simulink model "carsim_experiment_commai"  (R2017a)
settings: Solver=ode45  StartTime=0  StopTime=200  FixedStep=0.002  RelTol=1e-3  AbsTol=1e-6
PreLoadFcn:
  | addpath C:\MKZ
  | bus_definitions
libraries: Solver_SF x1
settings Model: ExtModeTrigMode=oneshot  ExtModeArmWhenConnect=off  Creator=ywata  LastModifiedBy=User
settings DataIOCC: SaveFormat=Array  SignalLoggingName=sigsOut
settings OptimizationCC: BlockReduction=off  BooleanDataType=off  LifeSpan=inf
settings DebuggingCC: SaveWithParameterizedLinksMsg=none  UnderspecifiedInitializationDetection=Classic  MergeDetectMultiDrivingBlocksExec=none  SignalResolutionControl=TryResolveAllWithWarning  MultiTaskDSMMsg=warning  MultiTaskCondExecSysMsg=none  FcnCallInpInsideContextMsg=warning  StateNameClashWarn=warning  SFUnexpectedBacktrackingDiag=warning  SFNoUnconditionalDefaultTransitionDiag=warning  SFExecutionAtInitializationDiag=none
settings HardwareCC: ProdBitPerPointer=32  ProdBitPerSizeT=32  ProdBitPerPtrDiffT=32  ProdLargestAtomicFloat=None  ProdIntDivRoundTo=Undefined  ProdEndianess=Unspecified  ProdWordSize=32  ProdHWDeviceType=32-bit Generic  TargetBitPerPointer=64  TargetBitPerSizeT=64  TargetBitPerPtrDiffT=64  TargetLongLongMode=on  TargetIntDivRoundTo=Zero  TargetEndianess=LittleEndian  TargetWordSize=64  TargetHWDeviceType=MATLAB Host  ProdEqTarget=off
settings ModelReferenceCC: UpdateModelReferenceTargets=Force  ModelReferenceNumInstancesAllowed=Single  PropagateSignalLabelsOutOfModel=off
settings ModelReferenceCC: ModelDependencies=|
  | lk_pcis_controller.m
  | road.m
settings RTWCC: TemplateMakefile=grt_vc.tmf
settings GRTTargetCC: TargetFcnLib=ansi_tfl_tmw.mat  TargetLangStandard=C89/C90 (ANSI)  GeneratePreprocessorConditionals=Disable all  CombineOutputUpdateFcns=off  GRTInterface=on
settings ConfigComp: CovMetricSettings=dw  CovHtmlReporting=on  CovSaveCumulativeToWorkspaceVar=on  CovSaveSingleToWorkspaceVar=on  CovExternalEMLEnable=off

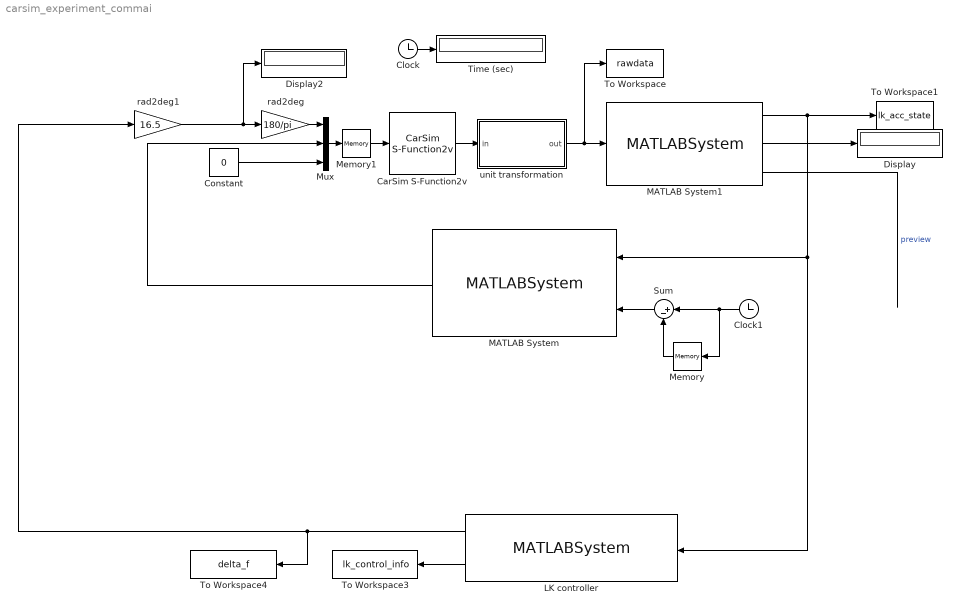
== system carsim_experiment_commai ==
  CarSim S-Function2v : Solver_SF/CarSim S-Function2v  Priority=1  VehicleCode=i_i  SIMFILE=simfile.sim
      settings: AttributesFormatString=Vehicle Code: %<VehicleCode>
  Clock : Clock
  Clock1 : Clock
  Constant : Constant  Value=0
  Display : Display
  Display2 : Display
  LK controller : MATLABSystem  System=lk_pcis_controller  M=1800  lf=1.2  lr=1.650  Caf=140000  Car=120000  Iz=3270.0  H_x=diag([1 0 0.5 0])  f_x=[0;0;0;0]  H_u=0.25  f_u=0  sol_opts=struct( 'DataType', 'double', 'MaxIter', 200, 'FeasibilityTol', 1e-6, 'IntegrityChecks', true )  SimulateUsing=Code generation
      mask Type: lk_pcis_controller
      mask Display:
      | disp('lk_pcis_controller');
      | port_label('input',1,'lk_acc_state');
      | port_label('output',1,'delta_f');
      | port_label('output',2,'control_info');
  MATLAB System : MATLABSystem  System=acc_pid_controller  mu_des=28/3.6  K_p=0.6*0.25  K_d=3*0.25*0.7/40  K_i=1.2*0.25/0.7  windup_reg=2  mem_length=20  max_throttle=0.3  SimulateUsing=Code generation
      mask Type: acc_pid_controller
      mask Display:
      | disp('acc_pid_controller');
      | port_label('input',1,'lk_acc_state');
      | port_label('input',2,'dt');
      | port_label('output',1,'throttle');
  MATLAB System1 : MATLABSystem  System=road  lat0=42.30095833  long0=-83.69758056  h0=0  pathfile=c:/mkz/mcity/carsim_mcity_outer_smooth.ascii  circular=0  N_path=3  N_interp=10  dt=0.1  compute_preview=true  SimulateUsing=Code generation
      mask Type: road
      mask Display:
      | disp('road');
      | port_label('input',1,'data');
      | port_label('output',1,'lk_acc_state');
      | port_label('output',2,'road_left');
      | port_label('output',3,'preview');
  Memory : Memory
  Memory1 : Memory  X0=[0;0;0]
  Mux : Mux  Inputs=3
  Sum : Sum  Inputs=|+-
  Time (sec) : Display
      settings: Format=bank  Decimation=100
  To Workspace : ToWorkspace  VariableName=rawdata  SaveFormat=Timeseries  SampleTime=-1
  To Workspace1 : ToWorkspace  VariableName=lk_acc_state  SaveFormat=Timeseries  SampleTime=-1
  To Workspace3 : ToWorkspace  VariableName=lk_control_info  SaveFormat=Timeseries  SampleTime=-1
  To Workspace4 : ToWorkspace  VariableName=delta_f  SaveFormat=Timeseries  SampleTime=-1
  rad2deg : Gain  Gain=180/pi
  rad2deg1 : Gain  Gain=16.5
  "unit transformation " : MATLAB Function  TreatAsAtomicUnit=on
  wires:
  Clock/1 -> Time (sec)/1
  LK controller/1 -> rad2deg1/1, To Workspace4/1
  LK controller/2 -> To Workspace3/1
  CarSim S-Function2v/1 -> "unit transformation "/1(in)
  Memory1/1 -> CarSim S-Function2v/1
  "unit transformation "/1(out) -> To Workspace/1, MATLAB System1/1
  rad2deg1/1 -> Display2/1, rad2deg/1
  rad2deg/1 -> Mux/1
  MATLAB System1/1 -> LK controller/1, MATLAB System/1, To Workspace1/1
  Mux/1 -> Memory1/1
  MATLAB System1/2 -> Display/1
  Clock1/1 -> Sum/1, Memory/1
  Sum/1 -> MATLAB System/2
  Memory/1 -> Sum/2
  MATLAB System/1 -> Mux/2
  Constant/1 -> Mux/3
  MATLAB System1/3 -> ?  "preview"

== matlab function carsim_experiment_commai/unit transformation  ==
  data: out output Bus: DataBus; in input
function out  = fcn(in)
    out.latitude = in(1);
    out.longitude = in(2);
    out.el = 0;
    out.Yaw = deg2rad(in(3));
    out.YawRate = deg2rad(in(4));
    out.Vx = in(5)/3.6;
    out.Vy = in(6)/3.6;
    out.x_gps_cg = in(7)/1000;
    out.y_gps_cg = in(8)/1000;
    out.steer_L1 = deg2rad(in(9));
    out.steer_R1 = deg2rad(in(10));
    out.Alpha_L1 = deg2rad(in(11));
    out.Alpha_R1 = deg2rad(in(12));
    out.Fy_L1 = in(13);
    out.Fy_R1 = in(14);
    out.Fz_L1 = in(15);
    out.Fz_R1 = in(16);
    out.Fx  = in(17) + in(18);
    out.Gear_CL  = in(19);
    out.RGear_Tr  = in(20);
    out.AV_Eng = in(21);
    out.Throttle = in(22);
    out.Throttle_Eng = in(23);
    out.M_EngOut = in(24);
    out.AVy_L1 = in(25);
    out.AVy_L2 = in(26);
    out.AVy_R1 = in(27);
    out.AVy_R2 = in(28);
    out.My_Dr_L1 = in(29);
    out.My_Dr_L2 = in(30);
    out.My_Dr_R1 = in(31);
    out.My_Dr_R2 = in(32);
    out.F_pedal = in(33);
    out.Bk_pedal = in(34);
